simulink model "teleop_simple"  (R2017a)
settings: Solver=VariableStepAuto  StartTime=0.0  StopTime=10.0  RelTol=1e-3
values from neighbouring files (symbols this model uses):
  Ki = 0    [bilat_teleop_time_delay_params.m]    (also in sampled_data_bilat_teleop_time_delay_params.m)
  Kp = 10000    [Oct12workspace.mat]    (also in Test_apparatus_simulation.m = pp; bilat_teleop_time_delay_params.m = 0; custom_sim.m = 100; ode45_sim.m = 100)
undefined symbols (not defined in the file or in its folder): bm, bs, Jm, Js, sigbuilder_block
settings Model: Creator=salou  LastModifiedBy=salou

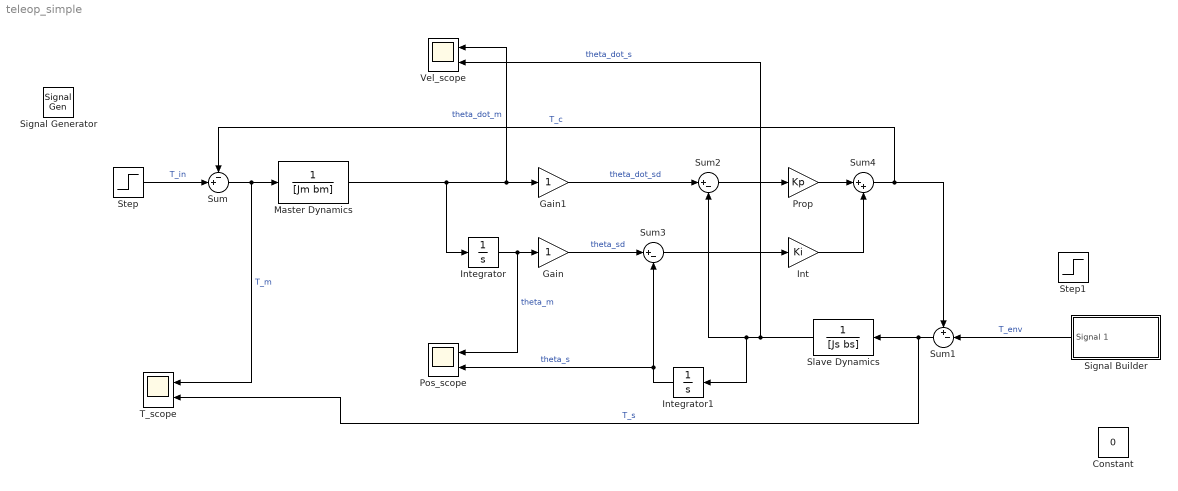
== system teleop_simple ==
  Constant : Constant  Value=0
  Gain : Gain
  Gain1 : Gain
  Int : Gain  Gain=Ki
  Integrator : Integrator
  Integrator1 : Integrator
  Master Dynamics : TransferFcn  Denominator=[Jm bm]
  Pos_scope : Scope  NumInputPorts=2
  Prop : Gain  Gain=Kp
  Signal Generator : SignalGenerator  WaveForm=square  Frequency=0.11
  Signal Builder : Subsystem  Tag=STV Subsys  LoadFcn=sigbuilder_block('load');  StartFcn=sigbuilder_block('start');  StopFcn=sigbuilder_block('stop');  ClipboardFcn=sigbuilder_block('clipboard');  mask(Sigbuilder block){tuvar=[0:10]}
      mask help: Simulink:masks:SigbuilderBlock_MD
      mask init:
      | if ~strcmp(get_param(bdroot(gcbh),'SimulationStatus'),'stopped') tuvar = sigbuilder_block('maskInit'); end
      settings: CopyFcn=sigbuilder_block('copy');  DeleteFcn=sigbuilder_block('delete');  ModelCloseFcn=sigbuilder_block('modelClose');  PreSaveFcn=sigbuilder_block('preSave');  PauseFcn=sigbuilder_block('pause');  ContinueFcn=sigbuilder_block('continue');  NameChangeFcn=sigbuilder_block('namechange');  OpenFcn=sigbuilder_block('open',[437.6 199.2 550.4 400 ]);  CloseFcn=sigbuilder_block('close');
      mask Display: plot(0, 0, 100, 100,[2, 2, 32, 32, 2], [68, 8, 8, 68, 68],[32, 2], [38, 38], [32, 19, 2],[53, 60, 44], [32, 17, 17, 2],[16, 16, 31, 31]);txt = getActiveGroup(gcbh);text(2, 100, txt,'verticalAlignment', 'top');
  Slave Dynamics : TransferFcn  Denominator=[Js bs]
  Step : Step  SampleTime=0
  Step1 : Step  Time=3  SampleTime=0
  Sum : Sum  Inputs=-+|
  Sum1 : Sum  Inputs=+-|
  Sum2 : Sum  Inputs=|+-
  Sum3 : Sum  Inputs=|+-
  Sum4 : Sum  Inputs=|++
  T_scope : Scope  NumInputPorts=2
  Vel_scope : Scope  NumInputPorts=2
  wires:
  Sum/1 -> T_scope/1, Master Dynamics/1  "T_m"
  Integrator/1 -> Pos_scope/1, Gain/1  "theta_m"
  Gain1/1 -> Sum2/1  "theta_dot_sd"
  Gain/1 -> Sum3/1  "theta_sd"
  Sum3/1 -> Int/1
  Sum2/1 -> Prop/1
  Prop/1 -> Sum4/1
  Int/1 -> Sum4/2
  Sum4/1 -> Sum/1, Sum1/1  "T_c"
  Step/1 -> Sum/2  "T_in"
  Signal Builder/1(Signal 1) -> Sum1/2  "T_env"
  Sum1/1 -> T_scope/2, Slave Dynamics/1  "T_s"
  Slave Dynamics/1 -> Vel_scope/2, Integrator1/1, Sum2/2  "theta_dot_s"
  Integrator1/1 -> Sum3/2, Pos_scope/2  "theta_s"
  Master Dynamics/1 -> Integrator/1, Vel_scope/1, Gain1/1  "theta_dot_m"

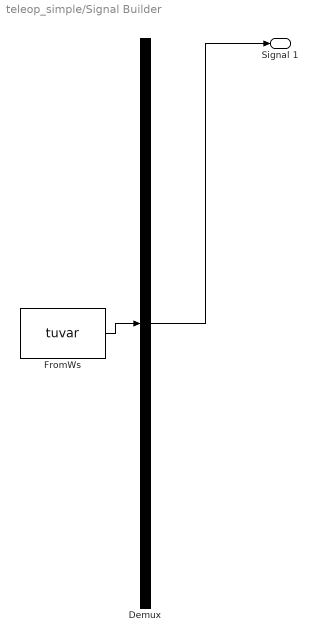
== system teleop_simple/Signal Builder ==
  Demux : Demux  Tag=STV Demux  Outputs=1
  FromWs : FromWorkspace  Tag=STV FromWs  VariableName=tuvar  SampleTime=0
      SigBuilderData=|
      | common.afterFinalStr = 'Extrapolate'
      | common.sampleTime = 0
      | dataSet.timeRange = [0 10]
      | dataSet.name = 'Group 1'
      | sbobj.Groups.Name = 'Group 1'
      | sbobj.Groups.Signals.Name = 'Signal 1'
      | sbobj.Groups.Signals.XData = [0 4 4 5 5 10]
      | sbobj.Groups.Signals.YData = [0 0 4 4 0 0]
  Signal 1 : Outport  Tag=STV Outport
  wires:
  Demux/1 -> Signal 1/1
  FromWs/1 -> Demux/1
